simulink model "JB_H10"  (R2025a)
settings: Solver=VariableStepAuto  StartTime=0.0  StopTime=2  MaxStep=2e-3  RelTol=1e-3
settings Model: Creator=Szalay  LastModifiedBy=Szalay

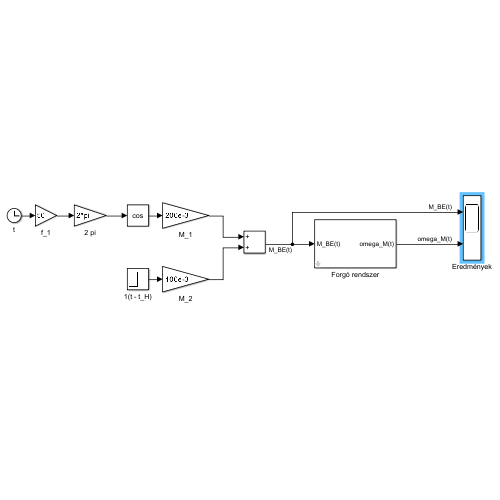
[thumbnail: Simulink's stored preview of the top-level diagram]
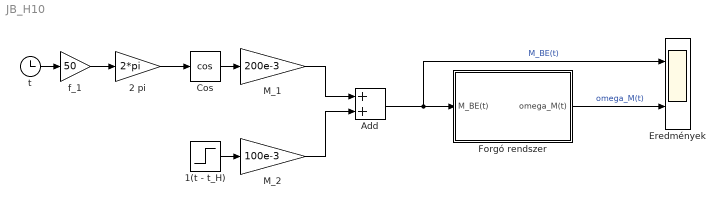
== system JB_H10 ==
  1(t - t_H) : Step  Time=1250e-3  SampleTime=0
  2 pi : Gain  Gain=2*pi
  Add : Sum
  Cos : Trigonometry  Operator=cos
  Eredmények : Scope  NumInputPorts=2
      settings: ActiveDisplayYMinimum=-40.260886899598482  ActiveDisplayYMaximum=240.13151259249329
  Forgó rendszer : Subsystem  mask(Forgó rendszer){J=500e-7, B=5e-4, omega_M0=100}
      mask prompts: J "Tehetetlenségi nyomaték (kg m^2)"; B "Forgási súrlódási együttható (N m s/rad)"; omega_M0 "Kezdeti szögsebesség (rad/s)"
      mask help: Súrlódó tengelyen forgó tömeg.
      mask DialogControl ParameterGroupVar Prompt: Rendszerparaméterek
      mask DialogControl Container3 Prompt: Kezdeti érték
  M_1 : Gain  Gain=200e-3
  M_2 : Gain  Gain=100e-3
  f_1 : Gain  Gain=50
  t : Clock
  wires:
  Add/1 -> Eredmények/1, Forgó rendszer/1(M_BE(t))  "M_BE(t)"
  M_1/1 -> Add/1
  Cos/1 -> M_1/1
  t/1 -> f_1/1
  f_1/1 -> 2 pi/1
  2 pi/1 -> Cos/1
  1(t - t_H)/1 -> M_2/1
  M_2/1 -> Add/2
  Forgó rendszer/1(omega_M(t)) -> Eredmények/2  "omega_M(t)"

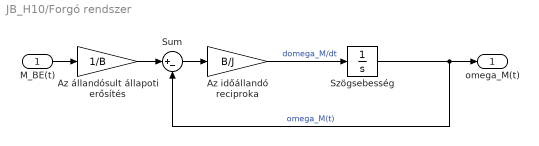
== system JB_H10/Forgó rendszer ==
  M_BE(t) : Inport
  Az időállandó reciproka : Gain  Gain=B/J
  Az állandósult állapoti erősítés : Gain  Gain=1/B
  Sum : Sum  Inputs=|+-
  Szögsebesség : Integrator  InitialCondition=omega_M0
  omega_M(t) : Outport
  wires:
  Szögsebesség/1 -> omega_M(t)/1, Sum/2  "omega_M(t)"
  Az állandósult állapoti erősítés/1 -> Sum/1
  Sum/1 -> Az időállandó reciproka/1
  Az időállandó reciproka/1 -> Szögsebesség/1  "domega_M/dt"
  M_BE(t)/1 -> Az állandósult állapoti erősítés/1
